simulink model "nominal_tracking_REALTIME"  (R2020b)
settings: Solver=ode45  StartTime=0.0  StopTime=5  FixedStep=0.001  RelTol=1e-3
undefined symbols (not defined in the file or in its folder): degs2rpm, denH1, DiscIntNeverNeededParam, N_u, N_x, National_Instruments, numH1, PCI, rpm2rads, sens, step_size
libraries: sldrtlib x3, simulink x2
settings Model: ExtModeTrigDuration=10000  Creator=utente  LastModifiedBy=tortoranic
settings DataIOCC: ReturnWorkspaceOutputs=off
settings RTWCC: Description=Simulink Desktop Real-Time  SystemTargetFile=sldrt.tlc  TemplateMakefile=sldrt.tmf  RTWCompilerOptimization=on
settings CodeAppCC: MaxIdLength=95
settings SimulinkDesktopRealTimeCC: TargetPreCompLibLocation=C:\Program Files\MATLAB\R2020b\toolbox\sldrt\lib\win64

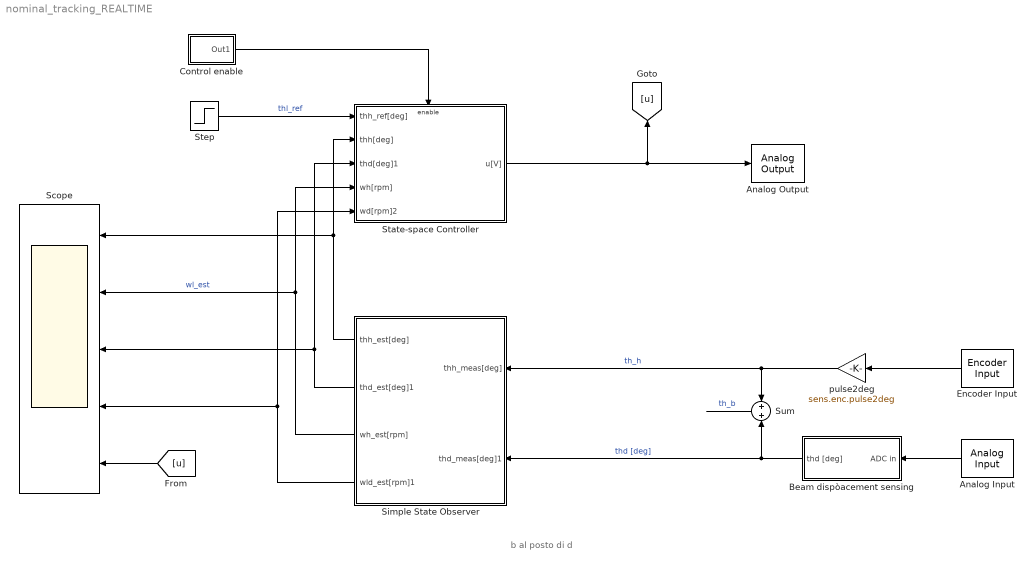
== system nominal_tracking_REALTIME ==
  note: b al posto di d
  Analog Input : sldrtlib/Analog Input  SampleTime=0.001  MaxMissedTicks=10  ShowMissedTicks=off  YieldWhenWaiting=off  DrvName=National_Instruments/PCI-6221  DrvAddress=4294967295  DrvOptions=[0 0 0 2 0]  Channels=[3 4]  RangeMode=1  VoltRange=2  DataType=1
      settings: AttributesFormatString=National Instruments\nPCI-6221 [auto]
  Analog Output : sldrtlib/Analog Output  SampleTime=0.001  MaxMissedTicks=10  ShowMissedTicks=off  YieldWhenWaiting=off  DrvName=National_Instruments/PCI-6221  DrvAddress=4294967295  DrvOptions=[0 0 0 2 0]  Channels=1  RangeMode=1  VoltRange=1  InitialValue=0  FinalValue=0
      settings: AttributesFormatString=National Instruments\nPCI-6221 [auto]
  Beam dispòacement sensing : Subsystem
  Control enable : Subsystem
  Encoder Input : sldrtlib/Encoder Input  SampleTime=0.001  MaxMissedTicks=10  ShowMissedTicks=off  YieldWhenWaiting=off  DrvName=National_Instruments/PCI-6221  DrvAddress=4294967295  DrvOptions=[0 0 0 2 0]  Channels=1  QuadMode=3  IndexPulse=1  InputFilter=Inf  DataType=1
      settings: AttributesFormatString=National Instruments\nPCI-6221 [auto]
  Scope : Scope  NumInputPorts=5
  Simple State Observer : Subsystem
  State-space Controller : Subsystem
  Step : Step  After=step_size  SampleTime=0.001
  Sum : Sum
  pulse2deg : Gain  Gain=sens.enc.pulse2deg
  wires:
  Step/1 -> State-space Controller/1(thh_ref[deg])  "thl_ref"
  Simple State Observer/1(thh_est[deg]) -> Scope/1, State-space Controller/2(thh[deg])
  Simple State Observer/3(wh_est[rpm]) -> Scope/2, State-space Controller/4(wh[rpm])  "wl_est"
  Encoder Input/1 -> pulse2deg/1
  pulse2deg/1 -> Simple State Observer/1(thh_meas[deg]), Sum/1  "th_h"
  State-space Controller/1(u[V]) -> Analog Output/1, [u]
  Simple State Observer/2(thd_est[deg]1) -> State-space Controller/3(thd[deg]1), Scope/3
  Simple State Observer/4(wld_est[rpm]1) -> State-space Controller/5(wd[rpm]2), Scope/4
  Analog Input/1 -> Beam dispòacement sensing/1(ADC in)
  Beam dispòacement sensing/1(thd [deg]) -> Simple State Observer/2(thd_meas[deg]1), Sum/2  "thd [deg]"
  Control enable/1(Out1) -> State-space Controller/Enable
  Sum/1 -> ?  "th_b"
  [u] -> Scope/5

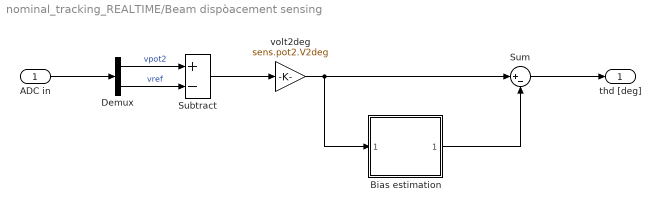
== system nominal_tracking_REALTIME/Beam dispòacement sensing ==
  ADC in : Inport
  Bias estimation : Subsystem
  Demux : Demux  Outputs=2
  Subtract : Sum  Inputs=+-
  Sum : Sum  Inputs=|+-
  volt2deg : Gain  Gain=sens.pot2.V2deg
  thd [deg] : Outport
  wires:
  Subtract/1 -> volt2deg/1
  Demux/1 -> Subtract/1  "vpot2"
  Demux/2 -> Subtract/2  "vref"
  ADC in/1 -> Demux/1
  volt2deg/1 -> Bias estimation/1(thd [deg]), Sum/1
  Bias estimation/1(thd_bias) -> Sum/2
  Sum/1 -> thd [deg]/1

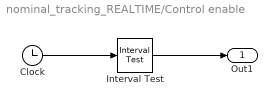
== system nominal_tracking_REALTIME/Control enable ==
  Clock : Clock
  Interval Test : simulink/Logic and Bit Operations/Interval Test  IntervalClosedRight=on  uplimit=60  IntervalClosedLeft=on  lowlimit=0.7  OutDataTypeStr=boolean
  Out1 : Outport
  wires:
  Clock/1 -> Interval Test/1
  Interval Test/1 -> Out1/1

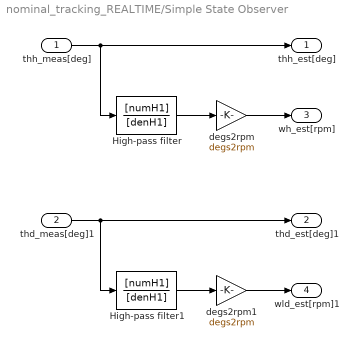
== system nominal_tracking_REALTIME/Simple State Observer ==
  thh_meas[deg] : Inport
  thd_meas[deg]1 : Inport  Port=2
  High-pass filter : TransferFcn  Numerator=[numH1]  Denominator=[denH1]
  High-pass filter1 : TransferFcn  Numerator=[numH1]  Denominator=[denH1]
  degs2rpm : Gain  Gain=degs2rpm
  degs2rpm1 : Gain  Gain=degs2rpm
  thh_est[deg] : Outport
  thd_est[deg]1 : Outport  Port=2
  wh_est[rpm] : Outport  Port=3
  wld_est[rpm]1 : Outport  Port=4
  wires:
  thh_meas[deg]/1 -> thh_est[deg]/1, High-pass filter/1
  High-pass filter/1 -> degs2rpm/1
  degs2rpm/1 -> wh_est[rpm]/1
  thd_meas[deg]1/1 -> thd_est[deg]1/1, High-pass filter1/1
  High-pass filter1/1 -> degs2rpm1/1
  degs2rpm1/1 -> wld_est[rpm]1/1

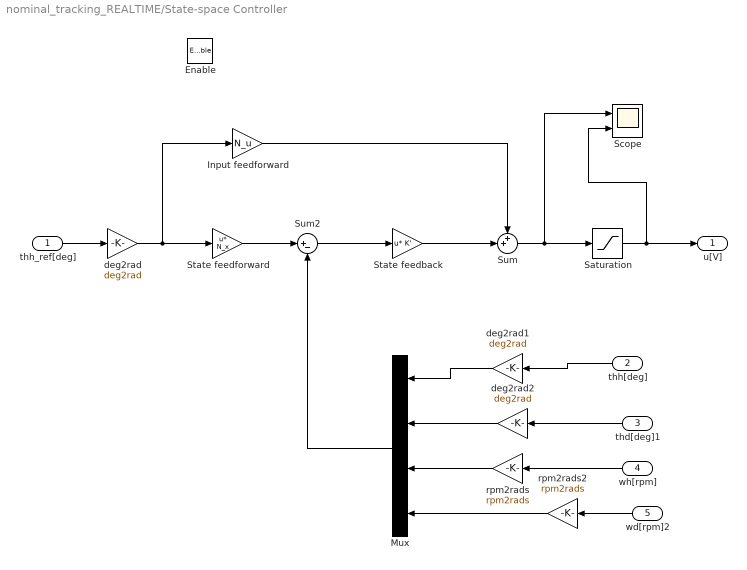
== system nominal_tracking_REALTIME/State-space Controller ==
  thh_ref[deg] : Inport
  thh[deg] : Inport  Port=2
  thd[deg]1 : Inport  Port=3
  wh[rpm] : Inport  Port=4
  wd[rpm]2 : Inport  Port=5
  Enable : EnablePort
  Input feedforward : Gain  Gain=N_u
  Mux : Mux
  Saturation : Saturate  UpperLimit=10  LowerLimit=-10
  Scope : Scope  NumInputPorts=2
  State feedback : Gain  Gain=K'  Multiplication=Matrix(u*K)
  "State feedforward\t" : Gain  Gain=N_x  Multiplication=Matrix(u*K)
  Sum : Sum  Inputs=++|
  Sum2 : Sum  Inputs=|+-
  deg2rad : Gain  Gain=deg2rad
  deg2rad1 : Gain  Gain=deg2rad
  deg2rad2 : Gain  Gain=deg2rad
  rpm2rads : Gain  Gain=rpm2rads
  rpm2rads2 : Gain  Gain=rpm2rads
  u[V] : Outport
  wires:
  thh_ref[deg]/1 -> deg2rad/1
  deg2rad/1 -> Input feedforward/1, "State feedforward\t"/1
  State feedback/1 -> Sum/2
  "State feedforward\t"/1 -> Sum2/1
  Sum2/1 -> State feedback/1
  Input feedforward/1 -> Sum/1
  Sum/1 -> Scope/1, Saturation/1
  Saturation/1 -> Scope/2, u[V]/1
  deg2rad1/1 -> Mux/1
  thh[deg]/1 -> deg2rad1/1
  wh[rpm]/1 -> rpm2rads/1
  Mux/1 -> Sum2/2
  rpm2rads/1 -> Mux/3
  thd[deg]1/1 -> deg2rad2/1
  wd[rpm]2/1 -> rpm2rads2/1
  deg2rad2/1 -> Mux/2
  rpm2rads2/1 -> Mux/4

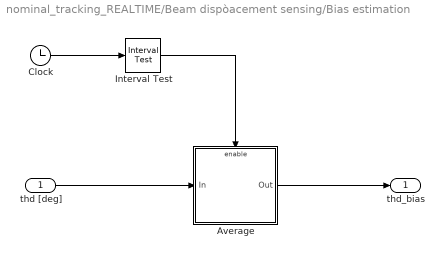
== system nominal_tracking_REALTIME/Beam dispòacement sensing/Bias estimation ==
  thd [deg] : Inport
  Average : Subsystem
  Clock : Clock
  Interval Test : simulink/Logic and Bit Operations/Interval Test  IntervalClosedRight=on  uplimit=0.7  IntervalClosedLeft=on  lowlimit=0.2  OutDataTypeStr=boolean
  thd_bias : Outport
  wires:
  Clock/1 -> Interval Test/1
  thd [deg]/1 -> Average/1(In)
  Average/1(Out) -> thd_bias/1
  Interval Test/1 -> Average/Enable

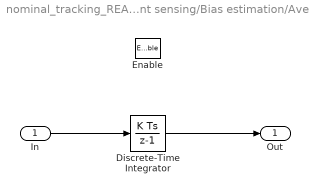
== system nominal_tracking_REALTIME/Beam dispòacement sensing/Bias estimation/Average ==
  In : Inport
  Enable : EnablePort
  Discrete-Time Integrator : DiscreteIntegrator  gainval=2.0  SampleTime=0.001  ICPrevOutput=DiscIntNeverNeededParam  ICPrevScaledInput=DiscIntNeverNeededParam
  Out : Outport
  wires:
  In/1 -> Discrete-Time Integrator/1
  Discrete-Time Integrator/1 -> Out/1
